simulink model "AVblock"  (R2016b)
settings: Solver=FixedStepDiscrete  StartTime=0.0  StopTime=10000  FixedStep=1  RelTol=1e-3
libraries: model_library x10
settings Model: Creator=dell  LastModifiedBy=dell

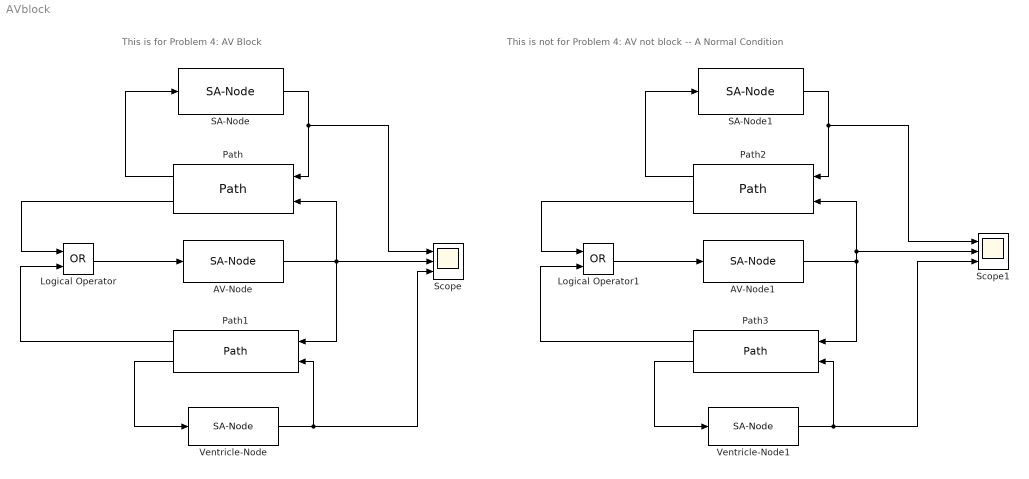
== system AVblock ==
  note: This is for Problem 4: AV Block
  note: This is not for Problem 4: AV not block -- A Normal Condition
  AV-Node : model_library/SA-Node
      link override Delay: InitialCondition=0  DelayLength=1  SampleTime=-1
      link override ERP_def: Value=500
      link override RRP_def: Value=0
      link override Rest_def: Value=1000
  AV-Node1 : model_library/SA-Node
      link override ERP_def: Value=500
      link override RRP_def: Value=0
      link override Rest_def: Value=1000
  Logical Operator : Logic  Operator=OR  AllPortsSameDT=off  OutDataTypeStr=boolean
  Logical Operator1 : Logic  Operator=OR  AllPortsSameDT=off  OutDataTypeStr=boolean
  Path : model_library/Path
      link override Tcond_def: Value=40
  Path1 : model_library/Path
      link override Tcond_def: Value=110
  Path2 : model_library/Path
      link override Tcond_def: Value=40
  Path3 : model_library/Path
      link override Tcond_def: Value=110
  SA-Node : model_library/SA-Node
      link override ERP_def: Value=200
      link override RRP_def: Value=0
      link override Rest_def: Value=200
  SA-Node1 : model_library/SA-Node
      link override ERP_def: Value=300
      link override RRP_def: Value=0
      link override Rest_def: Value=500
  Scope : Scope  NumInputPorts=3
  Scope1 : Scope  NumInputPorts=3
  Ventricle-Node : model_library/SA-Node
      link override ERP_def: Value=800
      link override Rest_def: Value=1200
  Ventricle-Node1 : model_library/SA-Node
      link override ERP_def: Value=800
      link override Rest_def: Value=1200
  wires:
  SA-Node/1 -> Scope/1, Path/1
  AV-Node/1 -> Path/2, Path1/1, Scope/2
  Path1/2 -> Ventricle-Node/1
  Ventricle-Node/1 -> Scope/3, Path1/2
  Path1/1 -> Logical Operator/2
  Path/2 -> Logical Operator/1
  Logical Operator/1 -> AV-Node/1
  Path/1 -> SA-Node/1
  SA-Node1/1 -> Scope1/1, Path2/1
  Path3/2 -> Ventricle-Node1/1
  Path3/1 -> Logical Operator1/2
  Path2/2 -> Logical Operator1/1
  Logical Operator1/1 -> AV-Node1/1
  Path2/1 -> SA-Node1/1
  Ventricle-Node1/1 -> Path3/2, Scope1/3
  AV-Node1/1 -> Path3/1, Scope1/2, Path2/2
